simulink model "MPC_feedforward_position"  (R2019b)
settings: Solver=ode45  StartTime=0.0  StopTime=10  RelTol=1e-3
undefined symbols (not defined in the file): force_multiplier, K, k_T, R, r, umpc
libraries: mblibv1 x13
settings Model: SimulationMode=accelerator  Creator=sansh  LastModifiedBy=lakshmi
settings DataIOCC: ReturnWorkspaceOutputs=off
settings DebuggingCC: ArithmeticOperatorsInVariantConditions=warning
settings SFSimCC: SimUseLocalCustomCode=off  CustomCodeUndefinedFunction=UseInterfaceOnly
settings RTWCC: RTWUseLocalCustomCode=off
settings CodeAppCC: StateflowObjectComments=on
settings SimscapeCC: SimscapeNormalizeSystem=off
settings SimMechanicsCC: VisDuringSimulation=on

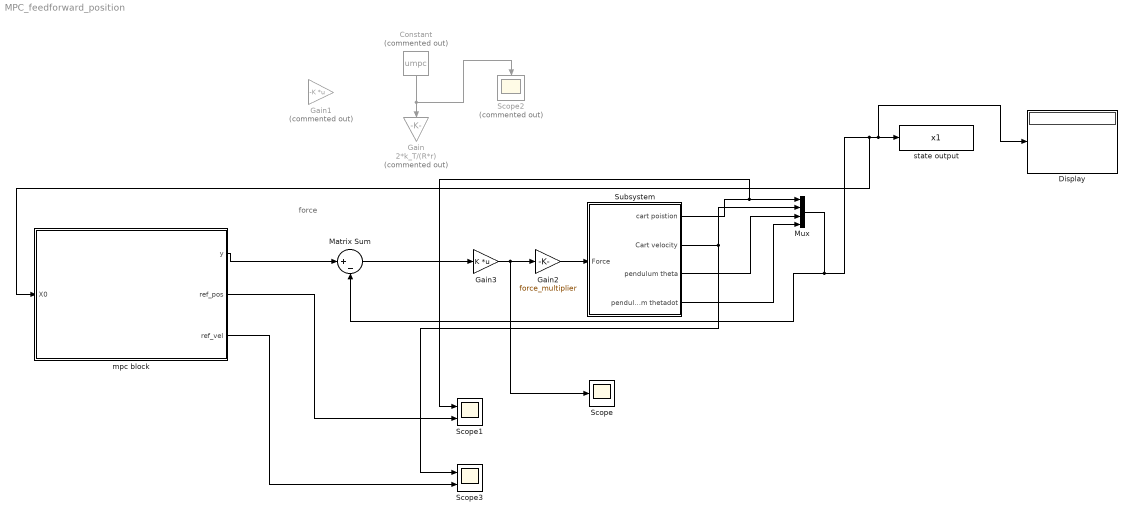
== system MPC_feedforward_position ==
  note: force
  Constant : Constant  Commented=on  Value=umpc
  Display : Display
  Gain : Gain  Commented=on  Gain=2*k_T/(R*r)
  Gain1 : Gain  Commented=on  Gain=-K  Multiplication=Matrix(K*u)
  Gain2 : Gain  Gain=force_multiplier
  Gain3 : Gain  Gain=K  Multiplication=Matrix(K*u)
  Matrix Sum : Sum  Inputs=|+-
  Mux : Mux
  Scope : Scope
  Scope1 : Scope  NumInputPorts=2
  Scope2 : Scope  Commented=on
  Scope3 : Scope  NumInputPorts=2
  Subsystem : Subsystem
  mpc block : MATLAB Function  TreatAsAtomicUnit=on
  state output : ToWorkspace  VariableName=x1  SampleTime=-1
  wires:
  Mux/1 -> Matrix Sum/2, mpc block/1(X0), Display/1, state output/1
  Constant/1 -> Scope2/1, Gain/1
  Subsystem/3(pendulum theta) -> Mux/3
  Gain2/1 -> Subsystem/1(Force)
  mpc block/1(y) -> Matrix Sum/1
  Matrix Sum/1 -> Gain3/1
  Gain3/1 -> Scope/1, Gain2/1
  mpc block/2(ref_pos) -> Scope1/2
  Subsystem/4(pendulum thetadot) -> Mux/4
  Subsystem/1(cart poistion) -> Scope1/1, Mux/1
  Subsystem/2(Cart velocity) -> Scope3/1, Mux/2
  mpc block/3(ref_vel) -> Scope3/2

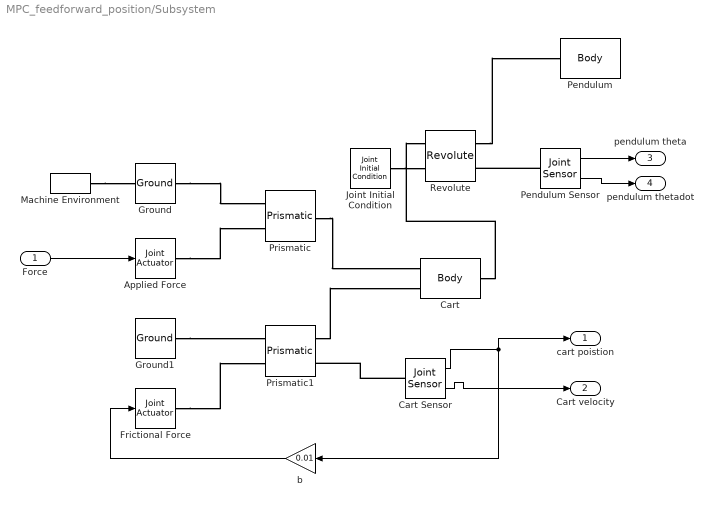
== system MPC_feedforward_position/Subsystem ==
  Force : Inport
  " Pendulum Sensor" : mblibv1/Sensors &  Actuators/Joint Sensor  UpdateFromCAD=off  PhysicalDomain=Mechanical  PortType=blob  Muxed=off  Pose=off  Angle=on  AngleUnits=rad  ArcVelocity=on  ArcVelocityUnits=rad/s  ArcAcceleration=off  ArcAccelerationUnits=deg/s^2  CoordPosition=on  CoordPositionUnits=m  Velocity=off  VelocityUnits=m/s  Acceleration=off  AccelerationUnits=m/s^2  Quaternion=on  QuaternionDT=off  QuaternionDDT=off  QuaternionUnits=off  OutputVector=[1]  ActiveIO=on  Width=2  DialogClass=MechanicalSensorBlock  Primitive=R1  Force=off  ForceUnits=N  Torque=off  TorqueUnits=N*m  ReferenceFrame=Absolute (World)  ReactionSensedSide=Base  ReactionReferenceFrame=Absolute (World)  ReactionForce=off  ReactionForceUnits=N  ReactionMoment=off  ReactionMomentUnits=N*m
      settings: SourceProductName=Simscape Multibody  SourceProductBaseCode=MS
  Applied Force : mblibv1/Sensors &  Actuators/Joint Actuator  UpdateFromCAD=off  PhysicalDomain=Mechanical  PortType=blob  ActuationStyle=Force  AngleUnits=deg  ArcVelocityUnits=deg/s  ArcAccelerationUnits=deg/s^2  CoordPositionUnits=m  VelocityUnits=m/s  AccelerationUnits=m/s^2  ForceUnits=N  TorqueUnits=N-m  ActiveIO=on  Width=1  DialogClass=MechanicalActuatorBlock  Primitive=P1  ReferenceFrame=Absolute (World)
      settings: SourceProductName=Simscape Multibody  SourceProductBaseCode=MS
  Cart : mblibv1/Bodies/Body  LConnTagsString=CS1|CS2  RConnTagsString=CS3  UpdateFromCAD=off  DialogClass=MechanicalBodyBlock  Mass=0.493  MassUnits=kg  InertiaUnits=kg*m^2  Inertia=eye(3)  Shape=Cylinder  ShapeDims=[1 1]  ShapeUnits=m  ShapeUse=false  Density=1  DensityUnits=kg/m^3  DensityUse=false  GraphicsMode=MACHINE_DEFAULT  BodyColorSelMode=COLORPALETTE  BodyColor=[0.501961;0.501961;0.501961]  AttachedToCS=CG  CG=Left$CG$[0 0 0]$WORLD$WORLD$m$[0 0 0]$Euler X-Y-Z$deg$WORLD$false$none  WorkingFrames=Left$CS1$[-0.04 0 0]$CG$CG$m$[0 0 0]$Euler X-Y-Z$deg$WORLD$true$none#Left$CS2$[0 0 0]$CG$CG$m$[0 0 0]$Euler X-Y-Z$deg$WORLD$true$none#Right$CS3$[0 0.035 0]$CG$CG$m$[0 0 0]$Euler X-Y-Z$deg$WORLD$true$none#Right$CS4$[-0.08 0.067 0]$CG$CG$m$[0 0 0]$Euler X-Y-Z$deg$WORLD$false$none#Right$CS5$[-0.08 -0.067 0]$CG$CG$m$[0 0 0]$Euler X-Y-Z$deg$WORLD$false$none#Right$CS6$[0.08 -0.067 0]$CG$CG$m$[0 0 0]$Euler X-Y-Z$deg$WORLD$false$none#Right$CS7$[0.08 0.067 0]$CG$CG$m$[0 0 0]$Euler X-Y-Z$deg$WORLD$false$none  CGPos=[0 0 0]  CGRot=[0 0 0]  CS0Pos=[]  CS0Rot=[]  CS1Pos=[-0.04 0 0]  CS1Rot=[0 0 0]  CS2Pos=[0 0 0]  CS2Rot=[0 0 0]  CS3Pos=[0 0.035 0]  CS3Rot=[0 0 0]  CS4Pos=[-0.08 0.067 0]  CS4Rot=[0 0 0]  CS5Pos=[-0.08 -0.067 0]  CS5Rot=[0 0 0]  CS6Pos=[0.08 -0.067 0]  CS6Rot=[0 0 0]  CS7Pos=[0.08 0.067 0]  CS7Rot=[0 0 0]  CS8Pos=[]  CS8Rot=[]  CS9Pos=[]  CS9Rot=[]  CS10Pos=[]  CS10Rot=[]  CS11Pos=[]  CS11Rot=[]  CS12Pos=[]  CS12Rot=[]  CS13Pos=[]  CS13Rot=[]  CS14Pos=[]  CS14Rot=[]  CS15Pos=[]  CS15Rot=[]  CS16Pos=[]  CS16Rot=[]  CS17Pos=[]  CS17Rot=[]  CS18Pos=[]  CS18Rot=[]  CS19Pos=[]  CS19Rot=[]  CS20Pos=[]  CS20Rot=[]
      settings: SourceProductName=Simscape Multibody  SourceProductBaseCode=MS
  Cart Sensor : mblibv1/Sensors &  Actuators/Joint Sensor  UpdateFromCAD=off  PhysicalDomain=Mechanical  PortType=blob  Muxed=off  Pose=off  Angle=on  AngleUnits=deg  ArcVelocity=off  ArcVelocityUnits=deg/s  ArcAcceleration=off  ArcAccelerationUnits=deg/s^2  CoordPosition=on  CoordPositionUnits=m  Velocity=on  VelocityUnits=m/s  Acceleration=off  AccelerationUnits=m/s^2  Quaternion=on  QuaternionDT=off  QuaternionDDT=off  QuaternionUnits=off  OutputVector=[1]  ActiveIO=on  Width=2  DialogClass=MechanicalSensorBlock  Primitive=P1  Force=off  ForceUnits=N  Torque=off  TorqueUnits=N*m  ReferenceFrame=Absolute (World)  ReactionSensedSide=Base  ReactionReferenceFrame=Absolute (World)  ReactionForce=off  ReactionForceUnits=N  ReactionMoment=off  ReactionMomentUnits=N*m
      settings: SourceProductName=Simscape Multibody  SourceProductBaseCode=MS
  Frictional Force : mblibv1/Sensors &  Actuators/Joint Actuator  UpdateFromCAD=off  PhysicalDomain=Mechanical  PortType=blob  ActuationStyle=Force  AngleUnits=deg  ArcVelocityUnits=deg/s  ArcAccelerationUnits=deg/s^2  CoordPositionUnits=m  VelocityUnits=m/s  AccelerationUnits=m/s^2  ForceUnits=N  TorqueUnits=N-m  ActiveIO=on  Width=1  DialogClass=MechanicalActuatorBlock  Primitive=P1  ReferenceFrame=Absolute (World)
      settings: SourceProductName=Simscape Multibody  SourceProductBaseCode=MS
  Ground : mblibv1/Bodies/Ground  UpdateFromCAD=off  LeftPortType=env  RightPortType=workingframe  PhysicalDomain=Mechanical  DialogClass=GroundBlock  CoordPosition=[0 0 0]  CoordPositionUnits=m  StateVectorMgrId=11  MachineId=[12 0]  ShowEnvPort=on  ParameterChecksum=[3479520630, 2024803054, 3212154210, 2990609347]  TopologyChecksum=[4245298806, 3648156196, 412969755, 138428968]
      settings: SourceProductName=Simscape Multibody  SourceProductBaseCode=MS
  Ground1 : mblibv1/Bodies/Ground  UpdateFromCAD=off  LeftPortType=env  RightPortType=workingframe  PhysicalDomain=Mechanical  DialogClass=GroundBlock  CoordPosition=[0 0 0]  CoordPositionUnits=m  StateVectorMgrId=-1  MachineId=[0 0]  ShowEnvPort=off  ParameterChecksum=[0 0 0 0]  TopologyChecksum=[0 0 0 0]
      settings: SourceProductName=Simscape Multibody  SourceProductBaseCode=MS
  Joint Initial Condition : mblibv1/Sensors &  Actuators/Joint Initial Condition  UpdateFromCAD=off  LeftPortType=blob  RightPortType=blob  PhysicalDomain=mechanical  DialogClass=InitialConditionBlock  InitialConditions=P1$false$0$m$deg$0$m/s$deg/s#P2$false$0$m$deg$0$m/s$deg/s#P3$false$0$m$deg$0$m/s$deg/s#R1$true$20$m$deg$0$m/s$deg/s#R2$false$0$m$deg$0$m/s$deg/s#R3$false$0$m$deg$0$m/s$deg/s#S$false$0$m$deg$0$m/s$deg/s  P1PIC=0  P1VIC=0  P2PIC=0  P2VIC=0  P3PIC=0  P3VIC=0  R1PIC=20  R1VIC=0  R2PIC=0  R2VIC=0  R3PIC=0  R3VIC=0  SPIC=0  SVIC=0
      settings: SourceProductName=Simscape Multibody  SourceProductBaseCode=MS
  Machine Environment : mblibv1/Bodies/Machine Environment  PortType=env  PhysicalDomain=Mechanical  DialogTemplateClass=MECH.MachineEnvironment  SyncWhenCopied=off  Gravity=[0 -9.81 0]  GravityUnits=m/s^2  GravityAsSignal=off  Dimensionality=Auto-detect  AnalysisType=Forward dynamics  LinearAssemblyTolerance=1e-3  LinearAssemblyToleranceUnits=m  AngularAssemblyTolerance=1e-3  AngularAssemblyToleranceUnits=rad  ConstraintSolverType=Stabilizing  ConstraintRelTolerance=1e-4  ConstraintAbsTolerance=1e-4  UseRobustSingularityHandling=off  RedundancyAnalysisToleranceType=Automatically select tolerance  RedundancyAnalysisTolerance=1e-14  StatePerturbationType=Fixed  PerturbationSize=1e-5  VisualizeMachine=on  BodyVisualizationType=Use model default body geometries  BodyColorSelMode=Use model default  DefaultBodyColor=[1 0 0]
      settings: SourceProductName=Simscape Multibody  SourceProductBaseCode=MS
  Pendulum : mblibv1/Bodies/Body  LConnTagsString=CS1  UpdateFromCAD=off  DialogClass=MechanicalBodyBlock  Mass=0.312  MassUnits=kg  InertiaUnits=kg*m^2  Inertia=0.00024*eye(3)  Shape=Cylinder  ShapeDims=[1 1]  ShapeUnits=m  ShapeUse=false  Density=1  DensityUnits=kg/m^3  DensityUse=false  GraphicsMode=MACHINE_DEFAULT  BodyColorSelMode=COLORPALETTE  BodyColor=[0.07451;0.62353;1]  AttachedToCS=CG  CG=Left$CG$[0 0.055 0]$CS1$CS1$m$[0 0 0]$Euler X-Y-Z$deg$WORLD$false$none  WorkingFrames=Left$CS1$[0 0 0]$Adjoining$Adjoining$m$[0 0 0]$Euler X-Y-Z$deg$WORLD$true$none#Right$CS2$[0.04 0 0]$CS1$CS1$m$[0 0 0]$Euler X-Y-Z$deg$WORLD$false$none#Right$CS3$[-0.04 0 0]$CS1$CS1$m$[0 0 0]$Euler X-Y-Z$deg$WORLD$false$none#Right$CS4$[-0.04 0.11 0]$CS1$CS1$m$[0 0 0]$Euler X-Y-Z$deg$WORLD$false$none#Right$CS5$[0.04 0.11 0]$CS1$CS1$m$[0 0 0]$Euler X-Y-Z$deg$WORLD$false$none  CGPos=[0 0.055 0]  CGRot=[0 0 0]  CS0Pos=[]  CS0Rot=[]  CS1Pos=[0 0 0]  CS1Rot=[0 0 0]  CS2Pos=[0.04 0 0]  CS2Rot=[0 0 0]  CS3Pos=[-0.04 0 0]  CS3Rot=[0 0 0]  CS4Pos=[-0.04 0.11 0]  CS4Rot=[0 0 0]  CS5Pos=[0.04 0.11 0]  CS5Rot=[0 0 0]  CS6Pos=[]  CS6Rot=[]  CS7Pos=[]  CS7Rot=[]  CS8Pos=[]  CS8Rot=[]  CS9Pos=[]  CS9Rot=[]  CS10Pos=[]  CS10Rot=[]  CS11Pos=[]  CS11Rot=[]  CS12Pos=[]  CS12Rot=[]  CS13Pos=[]  CS13Rot=[]  CS14Pos=[]  CS14Rot=[]  CS15Pos=[]  CS15Rot=[]  CS16Pos=[]  CS16Rot=[]  CS17Pos=[]  CS17Rot=[]  CS18Pos=[]  CS18Rot=[]  CS19Pos=[]  CS19Rot=[]  CS20Pos=[]  CS20Rot=[]
      settings: SourceProductName=Simscape Multibody  SourceProductBaseCode=MS
  Prismatic : mblibv1/Joints/Prismatic  LConnTagsString=__newl0|SA1  RConnTagsString=__newr0  UpdateFromCAD=off  NumSAPorts=1  CutJoint=off  MarkAsCut=off  Primitives=prismatic  PrimitiveProps=P1$World$[1 0 0]$prismatic  DialogClass=JointBlock  P1Axis=[1 0 0]
      settings: SourceProductName=Simscape Multibody  SourceProductBaseCode=MS
  Prismatic1 : mblibv1/Joints/Prismatic  LConnTagsString=__newl0|SA1  RConnTagsString=__newr0|SA1  UpdateFromCAD=off  NumSAPorts=2  CutJoint=off  MarkAsCut=off  Primitives=prismatic  PrimitiveProps=P1$World$[1 0 0]$prismatic  DialogClass=JointBlock  P1Axis=[1 0 0]
      settings: SourceProductName=Simscape Multibody  SourceProductBaseCode=MS
  Revolute : mblibv1/Joints/Revolute  LConnTagsString=__newl0|SA1  RConnTagsString=__newr0|SA1  UpdateFromCAD=off  NumSAPorts=2  CutJoint=off  MarkAsCut=off  Primitives=prismatic  PrimitiveProps=R1$World$[0 0 1]$revolute  DialogClass=JointBlock  R1Axis=[0 0 1]
      settings: SourceProductName=Simscape Multibody  SourceProductBaseCode=MS
  b : Gain  Gain=0.01
  cart poistion : Outport
  Cart velocity : Outport  Port=2
  pendulum theta : Outport  Port=3
  pendulum thetadot : Outport  Port=4
  wires:
  Force/1 -> Applied Force/1
  Cart Sensor/2 -> Cart velocity/1
  b/1 -> Frictional Force/1
  " Pendulum Sensor"/1 -> pendulum theta/1
  " Pendulum Sensor"/2 -> pendulum thetadot/1
  Cart Sensor/1 -> cart poistion/1, b/1
  connections:
  Revolute/RConn1 -- Pendulum/LConn1
  Joint Initial Condition/RConn1 -- Revolute/LConn2
  Cart/RConn1 -- Revolute/LConn1
  Machine Environment/RConn1 -- Ground/LConn1
  Prismatic1/RConn1 -- Cart/LConn2
  Ground1/RConn1 -- Prismatic1/LConn1
  Prismatic/RConn1 -- Cart/LConn1
  " Pendulum Sensor"/LConn1 -- Revolute/RConn2
  Cart Sensor/LConn1 -- Prismatic1/RConn2
  Applied Force/RConn1 -- Prismatic/LConn2
  Frictional Force/RConn1 -- Prismatic1/LConn2
  Ground/RConn1 -- Prismatic/LConn1

== matlab function MPC_feedforward_position/mpc block ==
  settings: updateMethod=DISCRETE
  data: X0 input; y output; ref_pos output; obj parameter; ref_vel output
function [y,ref_pos,ref_vel]= fcn(X0,obj)
    y = [0;0;0;0];
    ref_pos = 0;
    
    refbar = zeros(4*obj.N,1);
    X0bar = zeros(4*obj.N,1);
    persistent ii

    if isempty(ii)
        ii = 1;
    end
    
    coder.extrinsic('quadprog');
    for kk = 1:obj.N
        refbar(4*(kk-1)+1: 4*(kk)) = [obj.ref_X(ii+kk);(obj.ref_X(ii+kk)-X0(1))*0.1 ;0 ; 0];
        X0bar(4*(kk-1)+1: 4*(kk))= [X0(1);X0(2);X0(3);X0(4)];
    end

    
    %W = obj.W0 + [-obj.Nbar*X0bar;obj.Nbar*X0bar; -obj.Sx*X0bar; obj.Sx*X0bar];
    
    W = obj.W0 + [-obj.Nbar*X0bar;obj.Nbar*X0bar];
    f = refbar'*obj.Fr + X0bar'*obj.Fx;
    
    Z = quadprog(obj.H,f,obj.G,W,[],[],[],[],[])  %Here is the magic!
    
    y = Z(1:4);
    %ref_mpc = ref_mpc- X0;
    
    %u = obj.KT*obj.K*(ref_mpc);
    ii = ii+1;
    ref_pos = refbar(1);
    ref_vel = -refbar(2);
end
